simulink library "Lib_PFSys_GenericInverter_TMATS"  (R2019b)
settings: Solver=ode45  StartTime=0.0  StopTime=10.0  RelTol=1e-3  EnableMultiTasking=on
Description:
  | Thomas Modules
settings Model: Creator=jwchapm2  LastModifiedBy=mebell
settings DataIOCC: LimitDataPoints=on  SaveFormat=Array  ReturnWorkspaceOutputs=off
settings OptimizationCC: ExpressionDepthLimit=2147483647  LifeSpan=inf
settings DebuggingCC: UnderspecifiedInitializationDetection=Classic  MergeDetectMultiDrivingBlocksExec=none  SolverPrmCheckMsg=warning  StateNameClashWarn=warning  SFUnexpectedBacktrackingDiag=warning  SFNoUnconditionalDefaultTransitionDiag=warning  SFExecutionAtInitializationDiag=none  ArithmeticOperatorsInVariantConditions=warning
settings HardwareCC: ProdBitPerPointer=32  ProdBitPerSizeT=32  ProdBitPerPtrDiffT=32  ProdLargestAtomicFloat=None  ProdIntDivRoundTo=Undefined  ProdEndianess=Unspecified  ProdWordSize=32  ProdHWDeviceType=32-bit Generic
settings ModelReferenceCC: PropagateSignalLabelsOutOfModel=off
settings SFSimCC: SimUseLocalCustomCode=off  CustomCodeUndefinedFunction=UseInterfaceOnly
settings RTWCC: RTWUseLocalCustomCode=off
settings CodeAppCC: StateflowObjectComments=on
settings GRTTargetCC: TargetLangStandard=C89/C90 (ANSI)  GeneratePreprocessorConditionals=Disable all
settings ConfigComp: CovMetricSettings=dw  CovHtmlReporting=on  CovSaveCumulativeToWorkspaceVar=on  CovSaveSingleToWorkspaceVar=on  CovExternalEMLEnable=off

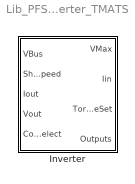
== system Lib_PFSys_GenericInverter_TMATS ==
  "Inverter " : Subsystem  mask(Inverter){Hz_to_V_M=22, X_C_VoltageVec_M=[0.0 0.1 1.0], Y_C_CurrentVec_M=[0.0 0.1 1.0], T_C_EffArray_M=[0.5 0.5 0.5; 0.5 1.0 1.0; 0.5 1.0 1.0], Pdis_M=1}
      mask prompts: Hz_to_V_M "Hz_to_V_M - Voltage/Flux Constant"; X_C_VoltageVec_M "X_C_VoltageVec_M - Efficiency Table Voltage Vector (X-axis)(nx1), V"; Y_C_CurrentVec_M "Y_C_CurrentVec_M - Efficiency Table Current Vector (Y-axis)(mx1), A"; T_C_EffArray_M "T_C_EffArray_M - Efficiency Table Values (Eff = f(i, V)(nxm)"; Pdis_M "Pdis_M - Constant Power Leaked/Dissipated, W"
      mask help:
      | This block represents a DC-to-AC inverter (for motor control). The block
      | produces an output voltage that scales with input frequency accoring to
      | the flux constant, Hz_to_V_M. The load is assumed to have no inductance,
      | and so we are assumed to operate with unity power factor. Converter
      | efficiency is specified via a lookup table that is a function of output
      | voltage and output current.

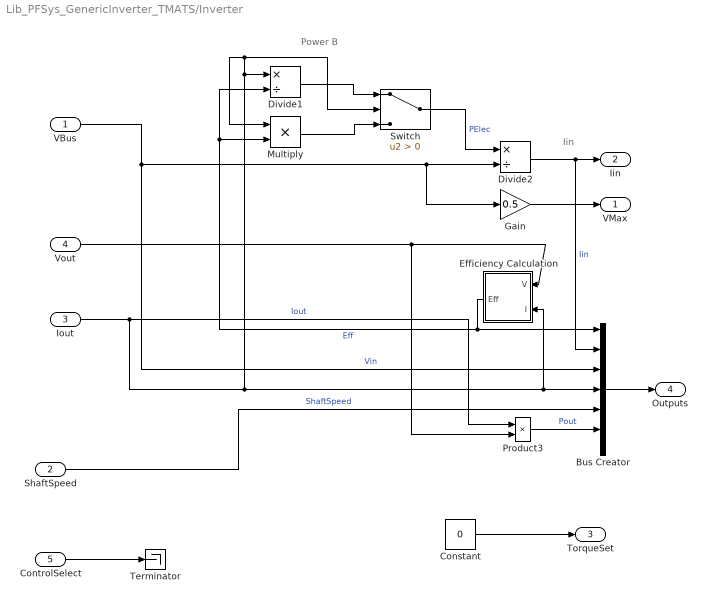
== system Lib_PFSys_GenericInverter_TMATS/Inverter  ==
  note: Iin
  note: Power B
  VBus : Inport
  "ShaftSpeed " : Inport  Port=2
  Iout : Inport  Port=3
  Vout : Inport  Port=4
  ControlSelect : Inport  Port=5
  Bus Creator : BusCreator  Inputs=7
  Constant : Constant  Value=0
  Divide1 : Product  Inputs=*/
  Divide2 : Product  Inputs=*/
  Efficiency Calculation : Subsystem
  Gain : Gain  Gain=0.5
  Multiply : Product
  Product3 : Product
  Switch : Switch  Criteria=u2 > Threshold
  Terminator : Terminator
  VMax : Outport  VectorParamsAs1DForOutWhenUnconnected=off
  Iin : Outport  Port=2  VectorParamsAs1DForOutWhenUnconnected=off
  TorqueSet : Outport  Port=3
  Outputs : Outport  Port=4  VectorParamsAs1DForOutWhenUnconnected=off
  wires:
  Product3/1 -> Bus Creator/6  "Pout"
  Bus Creator/1 -> Outputs/1
  "ShaftSpeed "/1 -> Bus Creator/5  "ShaftSpeed"
  VBus/1 -> Gain/1, Divide2/2, Bus Creator/3  "Vin"
  Iout/1 -> Product3/1, Bus Creator/4, Efficiency Calculation/2(I), Multiply/1, Switch/2, Divide1/1  "Iout"
  Gain/1 -> VMax/1
  Efficiency Calculation/1(Eff) -> Divide1/2, Multiply/2, Bus Creator/1  "Eff"
  Multiply/1 -> Switch/3
  Divide1/1 -> Switch/1
  Switch/1 -> Divide2/1  "PElec"
  Vout/1 -> Product3/2, Efficiency Calculation/1(V)
  Divide2/1 -> Bus Creator/2, Iin/1  "Iin"
  Constant/1 -> TorqueSet/1
  ControlSelect/1 -> Terminator/1

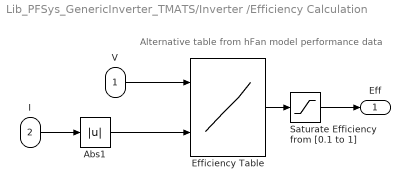
== system Lib_PFSys_GenericInverter_TMATS/Inverter /Efficiency Calculation ==
  note: Alternative table from hFan model performance data
  V : Inport
  I : Inport  Port=2
  Abs1 : Abs
  Efficiency Table : Lookup_n-D  BreakpointsForDimension1=X_C_VoltageVec_M  BreakpointsForDimension2=Y_C_CurrentVec_M  Table=T_C_EffArray_M  ExtrapMethod=Clip  InternalRulePriority=Speed  RndMeth=Simplest  InputSameDT=on
  Saturate Efficiency from [0.1 to 1] : Saturate  UpperLimit=1  LowerLimit=0.1
  Eff : Outport  VectorParamsAs1DForOutWhenUnconnected=off
  wires:
  Abs1/1 -> Efficiency Table/2
  Saturate Efficiency from [0.1 to 1]/1 -> Eff/1
  Efficiency Table/1 -> Saturate Efficiency from [0.1 to 1]/1
  I/1 -> Abs1/1
  V/1 -> Efficiency Table/1
